simulink model "PV_Cyber_Resilient_MVP"  (R2026a)
settings: Solver=ode3  StopTime=6.0  FixedStep=0.001
libraries: simulink x2
settings Model: Creator=sanmaestro7  LastModifiedBy=sanmaestro7

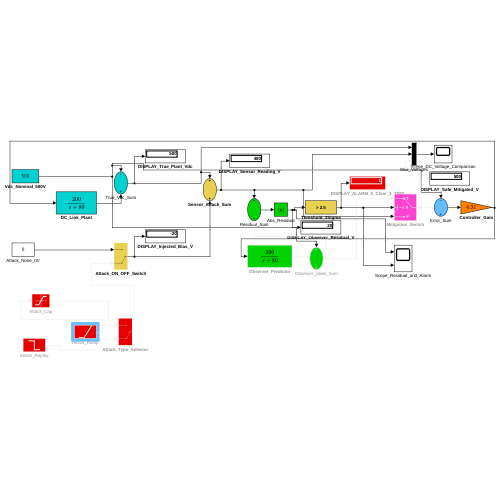
[thumbnail: Simulink's stored preview of the top-level diagram]
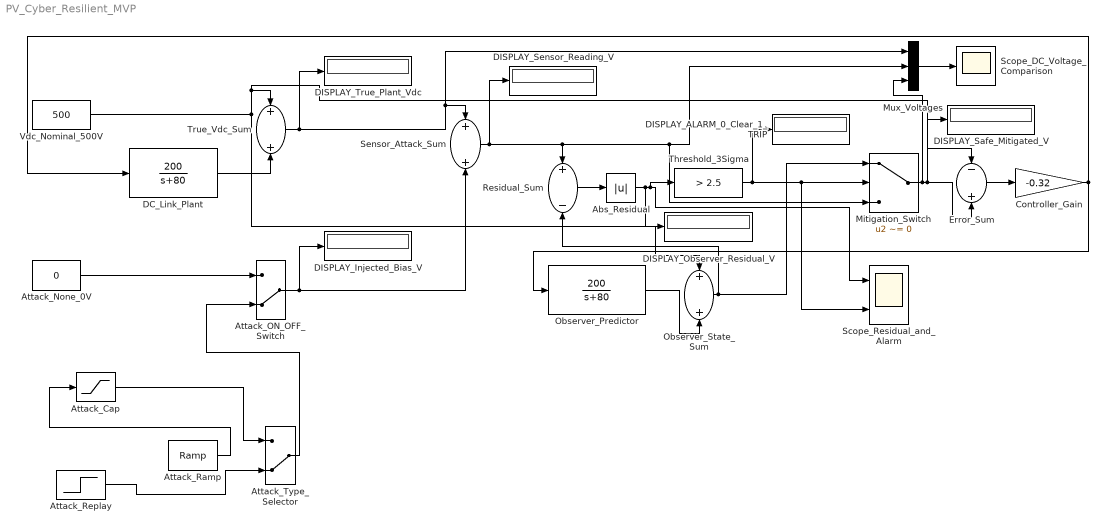
== system PV_Cyber_Resilient_MVP ==
  Abs_Residual : Abs  SaturateOnIntegerOverflow=off
  Attack_Cap : Saturate  UpperLimit=25  LowerLimit=0
  Attack_None_0V : Constant  Value=0
  Attack_ON_OFF_Switch : ManualSwitch  CurrentSetting=0
  Attack_Ramp : simulink/Sources/Ramp  slope=15  start=2.0  InitialOutput=0
  Attack_Replay : Step  Time=2.0  FinalValue=-20.0  SampleTime=0
  Attack_Type_Selector : ManualSwitch  CurrentSetting=0
  Controller_Gain : Gain  Gain=-0.32
  DC_Link_Plant : TransferFcn  Numerator=[200]  Denominator=[1 80]
  DISPLAY_ALARM_0_Clear_1_TRIP : Display
  DISPLAY_Injected_Bias_V : Display
  DISPLAY_Observer_Residual_V : Display
  DISPLAY_Safe_Mitigated_V : Display
  DISPLAY_Sensor_Reading_V : Display
  DISPLAY_True_Plant_Vdc : Display
  Error_Sum : Sum  Inputs=-+
  Mitigation_Switch : Switch  Criteria=u2 ~= 0  ZeroCross=off  SaturateOnIntegerOverflow=off  InputSameDT=off
  Mux_Voltages : Mux  Inputs=3
  Observer_Predictor : TransferFcn  Numerator=[200]  Denominator=[1 80]
  Observer_State_Sum : Sum
  Residual_Sum : Sum  Inputs=+-
  Scope_DC_Voltage_Comparison : Scope
      settings: ActiveDisplayYMinimum=477.5  ActiveDisplayYMaximum=502.5
  Scope_Residual_and_Alarm : Scope  NumInputPorts=2
      settings: ActiveDisplayYMinimum=-2.4999999999999996  ActiveDisplayYMaximum=22.5
  Sensor_Attack_Sum : Sum
  Threshold_3Sigma : simulink/Logic and Bit Operations/Compare To Constant  relop=>  const=2.5  OutDataTypeStr=boolean  ZeroCross=off
  True_Vdc_Sum : Sum
  Vdc_Nominal_500V : Constant  Value=500
  wires:
  Vdc_Nominal_500V/1 -> True_Vdc_Sum/1, Error_Sum/1, Observer_State_Sum/1
  DC_Link_Plant/1 -> True_Vdc_Sum/2
  True_Vdc_Sum/1 -> Sensor_Attack_Sum/1, Mux_Voltages/1, DISPLAY_True_Plant_Vdc/1
  Attack_Ramp/1 -> Attack_Cap/1
  Attack_Cap/1 -> Attack_Type_Selector/1
  Attack_Replay/1 -> Attack_Type_Selector/2
  Attack_None_0V/1 -> Attack_ON_OFF_Switch/1
  Attack_Type_Selector/1 -> Attack_ON_OFF_Switch/2
  Attack_ON_OFF_Switch/1 -> Sensor_Attack_Sum/2, DISPLAY_Injected_Bias_V/1
  Sensor_Attack_Sum/1 -> Mitigation_Switch/3, Mux_Voltages/2, Residual_Sum/1, DISPLAY_Sensor_Reading_V/1
  Observer_Predictor/1 -> Observer_State_Sum/2
  Observer_State_Sum/1 -> Residual_Sum/2, Mitigation_Switch/1
  Residual_Sum/1 -> Abs_Residual/1
  Abs_Residual/1 -> Threshold_3Sigma/1, Scope_Residual_and_Alarm/1, DISPLAY_Observer_Residual_V/1
  Threshold_3Sigma/1 -> Mitigation_Switch/2, Scope_Residual_and_Alarm/2, DISPLAY_ALARM_0_Clear_1_TRIP/1
  Mitigation_Switch/1 -> DISPLAY_Safe_Mitigated_V/1, Error_Sum/2, Mux_Voltages/3
  Error_Sum/1 -> Controller_Gain/1
  Controller_Gain/1 -> DC_Link_Plant/1, Observer_Predictor/1
  Mux_Voltages/1 -> Scope_DC_Voltage_Comparison/1
